simulink model "GCAWS"  (R2022a)
settings: Solver=FixedStepDiscrete  StartTime=0.0  StopTime=1  FixedStep=0.04  RelTol=1e-3
PreLoadFcn:
  | % Add Module Path
  | listing = dir;
  | if (contains([listing .name], 'TCAF')) && (contains([listing .name], 'MAP'))
  |     addpath('./TCAF', './MAP');
  |     addpath( genpath('./MAP') );
  | elseif (contains([listing .name], 'GCAWS.slx'))
  |     addpath('../TCAF', '../MAP');
  |     addpath( genpath('../MAP') );
  | else
  | end
  | 
  | % Add DataBus Path
  | load('BusStructureGCAWS.mat');
  | load('BusStructureWTPG.mat');
  | load('TRN\BusStructureTRN.mat');
InitFcn:
  | % Add Module Path
  | listing = dir;
  | if (contains([listing .name], 'TCAF')) && (contains([listing .name], 'MAP'))
  |     addpath('./TCAF', './MAP');
  |     addpath( genpath('./MAP') );
  | elseif (contains([listing .name], 'GCAWS.slx'))
  |     addpath('../TCAF', '../MAP');
  |     addpath( genpath('../MAP') );
  | else
  | end
  | 
  | % Add DataBus Path
  | load('BusStructureGCAWS.mat');
  | load('BusStructureWTPG.mat');
  | load('TRN\BusStructureTRN.mat');
StartFcn:
  | % Add Module Path
  | listing = dir;
  | if (contains([listing .name], 'TCAF')) && (contains([listing .name], 'MAP'))
  |     addpath('./TCAF', './MAP');
  |     addpath( genpath('./MAP') );
  | elseif (contains([listing .name], 'GCAWS.slx'))
  |     addpath('../TCAF', '../MAP');
  |     addpath( genpath('../MAP') );
  | else
  | end
  | 
  | % Add DataBus Path
  | load('BusStructureGCAWS.mat');
  | load('BusStructureWTPG.mat');
  | load('TRN\BusStructureTRN.mat');
values from neighbouring files (symbols this model uses):
  isFeasible = logsout{idx_WTPGDatapump}.Values.isFeasible.Data(ii,:)    [WTPG_SIM_AFTERPLOT.m]
undefined symbols (not defined in the file or in its folder): accNED, C_b_n, collisionWarning, collisionWarningValid, gOnsetRateWrap, lla, maxFlightPathAngleWrap, offObstructionMap, offTerrainMap, params, paramSelectedValid, pullUpGWrap, reactionTimeWrap, rollRateWrap, selectedWrap, statusCode, timeToGoToPullUp, velNED
libraries: hdlsllib x15, simulink x2
(part 1 of 2)
settings Model: Creator=ASCL  LastModifiedBy=ASCL
settings DataIOCC: SaveOutput=off  SignalLogging=off  DSMLogging=off  SaveTime=off  ReturnWorkspaceOutputs=off
settings OptimizationCC: BlockReduction=off  DefaultParameterBehavior=Inlined  UseDivisionForNetSlopeComputation=on  GainParamInheritBuiltInType=on  UseFloatMulNetSlope=on  ExpressionFolding=off  PassReuseOutputArgsAs=Individual arguments  ZeroExternalMemoryAtStartup=off  ZeroInternalMemoryAtStartup=off  EfficientFloat2IntCast=on  LifeSpan=inf  OptimizeBlockOrder=speed  DifferentSizesBufferReuse=on  EfficientTunableParamExpr=on
settings DebuggingCC: SignalInfNanChecking=warning  ReadBeforeWriteMsg=EnableAllAsError  WriteAfterWriteMsg=EnableAllAsError  WriteAfterReadMsg=EnableAllAsError  IntegerOverflowMsg=error  ParameterTunabilityLossMsg=error  UniqueDataStoreMsg=error  AssertControl=DisableAll  NonBusSignalsTreatedAsBus=error  SFInvalidInputDataAccessInChartInitDiag=error  SFTransitionOutsideNaturalParentDiag=error  SFUnreachableExecutionPathDiag=error  SFUndirectedBroadcastEventsDiag=error  IntegerSaturationMsg=error
settings HardwareCC: ProdBitPerPointer=32  ProdBitPerSizeT=32  ProdBitPerPtrDiffT=32  ProdLargestAtomicInteger=Long  ProdLargestAtomicFloat=Double  ProdEndianess=BigEndian  ProdWordSize=32  ProdLongLongMode=on  ProdHWDeviceType=Freescale->MPC83xx
settings ModelReferenceCC: ModelReferenceNumInstancesAllowed=Single
settings SFSimCC: SimCustomHeaderCode="#include \"MAP.h\""  SimUserSources=MAP.c  SimUserLibraries=WS2_32.LIB  CompileTimeRecursionLimit=0  EnableRuntimeRecursion=off  MATLABDynamicMemAlloc=off
settings RTWCC: SystemTargetFile=ert.tlc  TemplateMakefile=ert_default_tmf  GenerateReport=on  RTWUseSimCustomCode=on  CustomHeaderCode="#include \"MAP.h\""  CustomSource=MAP.c  CustomLibrary=WS2_32.LIB  BuildConfiguration=Faster Runs  IncludeHyperlinkInReport=on  LaunchReport=on  GenerateTraceInfo=on  GenerateTraceReport=on  GenerateTraceReportSl=on  GenerateTraceReportSf=on  GenerateTraceReportEml=on  GenerateCodeMetricsReport=on
settings CodeAppCC: ForceParamTrailComments=on  IgnoreCustomStorageClasses=off  OperatorAnnotations=on  SimulinkDataObjDesc=on  SFDataObjDesc=on  MATLABFcnDesc=on  InsertBlockDesc=on  StateflowObjectComments=on  MATLABSourceComments=on  EnableCustomComments=on  InlinedPrmAccess=Macros  ReqsInCode=on
settings ERTTargetCC: TargetLangStandard=C99 (ISO)  UtilityFuncGeneration=Shared location  GenerateSampleERTMain=on  IncludeMdlTerminateFcn=off  CombineSignalStateStructs=on  SuppressErrorStatus=on  SupportAbsoluteTime=off  SupportNonFinite=off  SupportComplex=off  SupportVariableSizeSignals=on  ParenthesesLevel=Standards  CastingMode=Standards  GenerateSharedConstants=off  InlinedParameterPlacement=NonHierarchical  ERTCustomFileTemplate=example_file_process.tlc  RateTransitionBlockCode=Function  PreserveIfCondition=on  ConvertIfToSwitch=off  EnableSignedLeftShifts=off  EnableSignedRightShifts=off

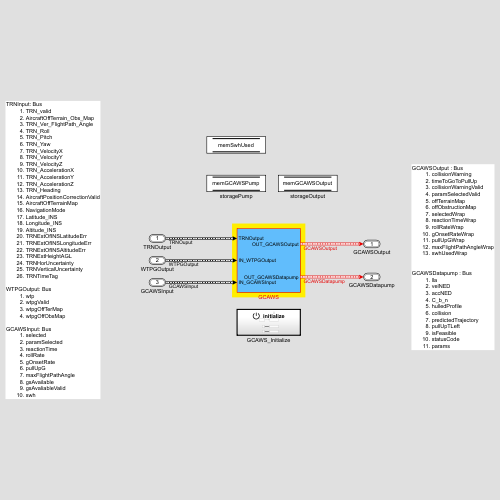
[thumbnail: Simulink's stored preview of the top-level diagram]
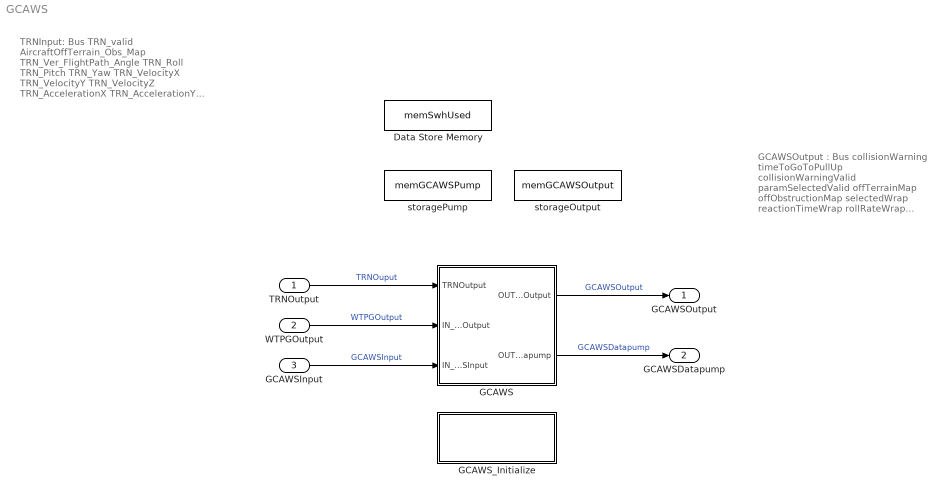
== system GCAWS ==
  note: TRNInput: Bus
      | TRN_valid
      | AircraftOffTerrain_Obs_Map
      | TRN_Ver_FlightPath_Angle
      | TRN_Roll
      | TRN_Pitch
      | TRN_Yaw
      | TRN_VelocityX
      | TRN_VelocityY
      | TRN_VelocityZ
      | TRN_AccelerationX
      | TRN_AccelerationY
      | TRN_AccelerationZ
      | TRN_Heading
      | AircraftPositionCorrectionValid
      | AircraftOffTerrainMap
      | NavigationMode
      | Latitude_INS
      | Longitude_INS
      | Altitude_INS
      | TRNEstOfINSLatitudeErr
      | TRNEstOfINSLongitudeErr
      | TRNEstOfINSAltitudeErr
      | TRNEstHeightAGL
      | TRNHorUncertainty
      | TRNVerticalUncertainty
      | TRNTimeTag
      |
      | WTPGOutput: Bus
      | wtp
      | wtpgValid
      | wtpgOffTerMap
      | wtpgOffObsMap
      |
      | GCAWSInput: Bus
      | selected
      | paramSelected
      | reactionTime
      | rollRate
      | gOnsetRate
      | pullUpG
      | maxFlightPathAngle
      | gsAvailable
      | gsAvaliableValid
      | swh
  note: GCAWSOutput : Bus
      | collisionWarning
      | timeToGoToPullUp
      | collisionWarningValid
      | paramSelectedValid
      | offTerrainMap
      | offObstructionMap
      | selectedWrap
      | reactionTimeWrap
      | rollRateWrap
      | gOnsetRateWrap
      | pullUpGWrap
      | maxFlightPathAngleWrap
      | swhUsedWrap
      |
      | GCAWSDatapump : Bus
      | lla
      | velNED
      | accNED
      | C_b_n
      | hulledProfile
      | collision
      | predictedTrajectory
      | pullUpTLeft
      | isFeasible
      | statusCode
      | params
  TRNOutput : Inport  OutDataTypeStr=Bus: TRNOutput  Interpolate=off  BusOutputAsStruct=on
  WTPGOutput : Inport  Port=2  OutDataTypeStr=Bus: WTPGOutput  Interpolate=off  BusOutputAsStruct=on
  GCAWSInput : Inport  Port=3  OutDataTypeStr=Bus: GCAWSInput  Interpolate=off  BusOutputAsStruct=on
  Data Store Memory : DataStoreMemory  DataStoreName=memSwhUsed  WriteAfterWriteMsg=warning  ShowAdditionalParam=off  OutDataTypeStr=single
  GCAWS : Subsystem
      mask init:
      | % latGPS = double(0);
      | % lonGPS = double(0);
      | % altGPS = double(0);
      | % velEGPS = double(0);
      | % velNGPS = double(0);
      | % velUGPS = double(0);
      | % notValidGPS = boolean(0);
      | % notAvaildINS = boolean(0);
      | % velUINS = double(0);
      | % velVINS = double(0);
      | % velWINS = double(0);
      | % rollINS = double(0);
      | % pitchINS = double(0);
      | % hgdINS = double(0);
      | % accXINS = double(0);
      | % accYINS = double(0);
      | % accZINS = double(0);
      | % activated = boolean(0);
      | % reactionT = uint16(0);
      | % pullUpG = uint16(0);
      | % rollRate = uint16(0);
      | % gOnsetRate = uint16(0);
      | % maxGamma = uint16(0);
      | % setWarnH = double(0);
      | % obsWarningTime = uint16(1);
      | % wiresWarningTime = uint16(1);
      | % latErrOfINS = double(0);
      | % lonErrOfINS = double(0);
      | % altErrorofINS = uint16(0);
      | % heightEstOfTRN = uint16(0);
      | % horUncertaintyOfTRN = double(0);
      | % verUncertaintyOfTRN = double(0);
  GCAWS_Initialize : Subsystem  TreatAsAtomicUnit=on
  storageOutput : DataStoreMemory  DataStoreName=memGCAWSOutput  WriteAfterWriteMsg=warning  WriteAfterReadMsg=warning  VectorParams1D=off  ShowAdditionalParam=off  OutDataTypeStr=Bus: GCAWSOutput
      settings: LockScale=on
  storagePump : DataStoreMemory  DataStoreName=memGCAWSPump  WriteAfterWriteMsg=warning  WriteAfterReadMsg=warning  VectorParams1D=off  ShowAdditionalParam=off  OutDataTypeStr=Bus: GCAWSDatapump
      settings: LockScale=on
  GCAWSOutput : Outport  OutDataTypeStr=Bus: GCAWSOutput  VectorParamsAs1DForOutWhenUnconnected=off  BusOutputAsStruct=on
  GCAWSDatapump : Outport  Port=2  OutDataTypeStr=Bus: GCAWSDatapump  VectorParamsAs1DForOutWhenUnconnected=off  BusOutputAsStruct=on
  wires:
  GCAWS/1(OUT_GCAWSOutput) -> GCAWSOutput/1  "GCAWSOutput"
  GCAWS/2(OUT_GCAWSDatapump) -> GCAWSDatapump/1  "GCAWSDatapump"
  GCAWSInput/1 -> GCAWS/3(IN_GCAWSInput)  "GCAWSInput"
  TRNOutput/1 -> GCAWS/1(TRNOutput)  "TRNOuput"
  WTPGOutput/1 -> GCAWS/2(IN_WTPGOutput)  "WTPGOutput"

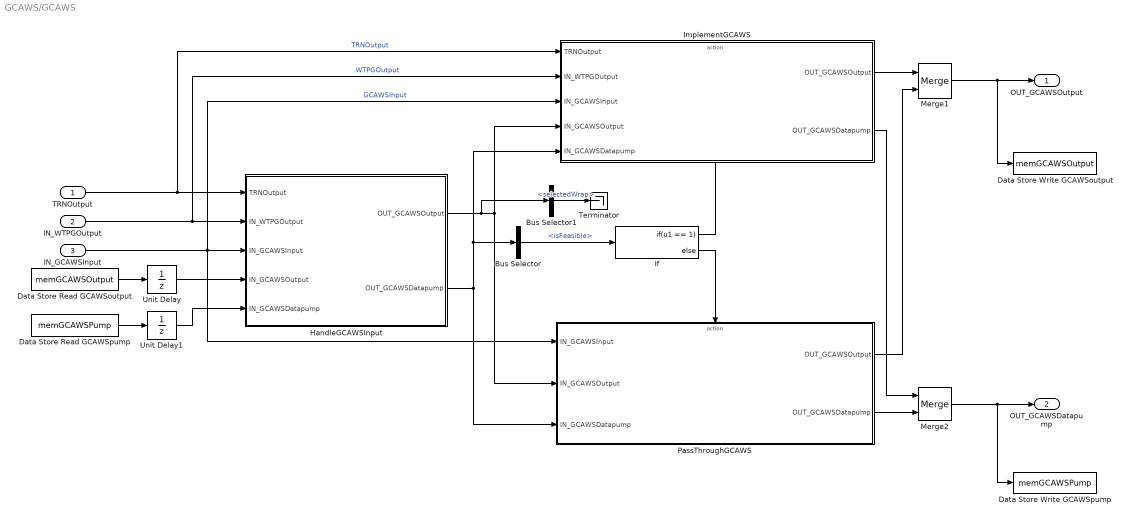
== system GCAWS/GCAWS ==
  TRNOutput : Inport  OutDataTypeStr=Bus: TRNOutput  BusOutputAsStruct=on
  IN_WTPGOutput : Inport  Port=2  OutDataTypeStr=Bus: WTPGOutput
  IN_GCAWSInput : Inport  Port=3  OutDataTypeStr=Bus: GCAWSInput
  Bus Selector : BusSelector  OutputSignals=isFeasible
  Bus Selector1 : BusSelector  OutputSignals=selectedWrap
  Data Store Read GCAWSoutput : DataStoreRead  DataStoreName=memGCAWSOutput  IndexOptions=Index vector (dialog)  Indices=1  OutputSizes=1
  Data Store Read GCAWSpump : DataStoreRead  DataStoreName=memGCAWSPump  IndexOptions=Index vector (dialog)  Indices=1  OutputSizes=1
  Data Store Write GCAWSoutput : DataStoreWrite  DataStoreName=memGCAWSOutput  IndexOptions=Index vector (dialog)  Indices=1  OutputSizes=1
  Data Store Write GCAWSpump : DataStoreWrite  DataStoreName=memGCAWSPump  IndexOptions=Index vector (dialog)  Indices=1  OutputSizes=1
  HandleGCAWSInput : Subsystem  TreatAsAtomicUnit=on
      settings: RTWSystemCode=Nonreusable function  RTWFcnNameOpts=Use subsystem name
  If : If  IfExpression=u1 == 1
  ImplementGCAWS : Subsystem  TreatAsAtomicUnit=on
      settings: RTWSystemCode=Nonreusable function  RTWFcnNameOpts=Use subsystem name
  Merge1 : Merge
  Merge2 : Merge
  PassThroughGCAWS : Subsystem  TreatAsAtomicUnit=on
      settings: RTWSystemCode=Nonreusable function  RTWFcnNameOpts=Use subsystem name
  Terminator : Terminator
  Unit Delay : UnitDelay  SampleTime=-1  HasFrameUpgradeWarning=on
  Unit Delay1 : UnitDelay  SampleTime=-1  HasFrameUpgradeWarning=on
  OUT_GCAWSOutput : Outport  OutDataTypeStr=Bus: GCAWSOutput  VectorParamsAs1DForOutWhenUnconnected=off
  OUT_GCAWSDatapump : Outport  Port=2  OutDataTypeStr=Bus: GCAWSDatapump  VectorParamsAs1DForOutWhenUnconnected=off
  wires:
  IN_GCAWSInput/1 -> ImplementGCAWS/3(IN_GCAWSInput), PassThroughGCAWS/1(IN_GCAWSInput), HandleGCAWSInput/3(IN_GCAWSInput)  "GCAWSInput"
  Merge1/1 -> Data Store Write GCAWSoutput/1, OUT_GCAWSOutput/1
  HandleGCAWSInput/1(OUT_GCAWSOutput) -> Bus Selector1/1, ImplementGCAWS/4(IN_GCAWSOutput), PassThroughGCAWS/2(IN_GCAWSOutput)
  HandleGCAWSInput/2(OUT_GCAWSDatapump) -> Bus Selector/1, ImplementGCAWS/5(IN_GCAWSDatapump), PassThroughGCAWS/3(IN_GCAWSDatapump)
  ImplementGCAWS/1(OUT_GCAWSOutput) -> Merge1/1
  PassThroughGCAWS/1(OUT_GCAWSOutput) -> Merge1/2
  PassThroughGCAWS/2(OUT_GCAWSDatapump) -> Merge2/2
  ImplementGCAWS/2(OUT_GCAWSDatapump) -> Merge2/1
  Merge2/1 -> OUT_GCAWSDatapump/1, Data Store Write GCAWSpump/1
  If/2 -> PassThroughGCAWS/Action
  If/1 -> ImplementGCAWS/Action
  IN_WTPGOutput/1 -> ImplementGCAWS/2(IN_WTPGOutput), HandleGCAWSInput/2(IN_WTPGOutput)  "WTPGOutput"
  TRNOutput/1 -> ImplementGCAWS/1(TRNOutput), HandleGCAWSInput/1(TRNOutput)  "TRNOutput"
  Bus Selector/1 -> If/1  "<isFeasible>"
  Data Store Read GCAWSoutput/1 -> Unit Delay/1
  Data Store Read GCAWSpump/1 -> Unit Delay1/1
  Unit Delay/1 -> HandleGCAWSInput/4(IN_GCAWSOutput)
  Unit Delay1/1 -> HandleGCAWSInput/5(IN_GCAWSDatapump)
  Bus Selector1/1 -> Terminator/1  "<selectedWrap>"

== system GCAWS/GCAWS_Initialize ==
  Constant : Constant  Value=[0, ]  OutDataTypeStr=Bus: GCAWSOutput
  Constant1 : Constant  Value=[0, ]  OutDataTypeStr=Bus: GCAWSDatapump
  Constant_single : Constant  Value=single(15.24)  OutDataTypeStr=single
  Data Store Write : DataStoreWrite  DataStoreName=memSwhUsed  IndexOptions=Index vector (dialog)  Indices=1  OutputSizes=1
  Data Store Write1 : DataStoreWrite  DataStoreName=memGCAWSPump  IndexOptions=Index vector (dialog)  Indices=1  OutputSizes=1
  Data Store Write2 : DataStoreWrite  DataStoreName=memGCAWSOutput  IndexOptions=Index vector (dialog)  Indices=1  OutputSizes=1
  Event Listener : EventListener  DisableCoverage=on  EventName=reset
  wires:
  Constant/1 -> Data Store Write2/1
  Constant_single/1 -> Data Store Write/1
  Constant1/1 -> Data Store Write1/1

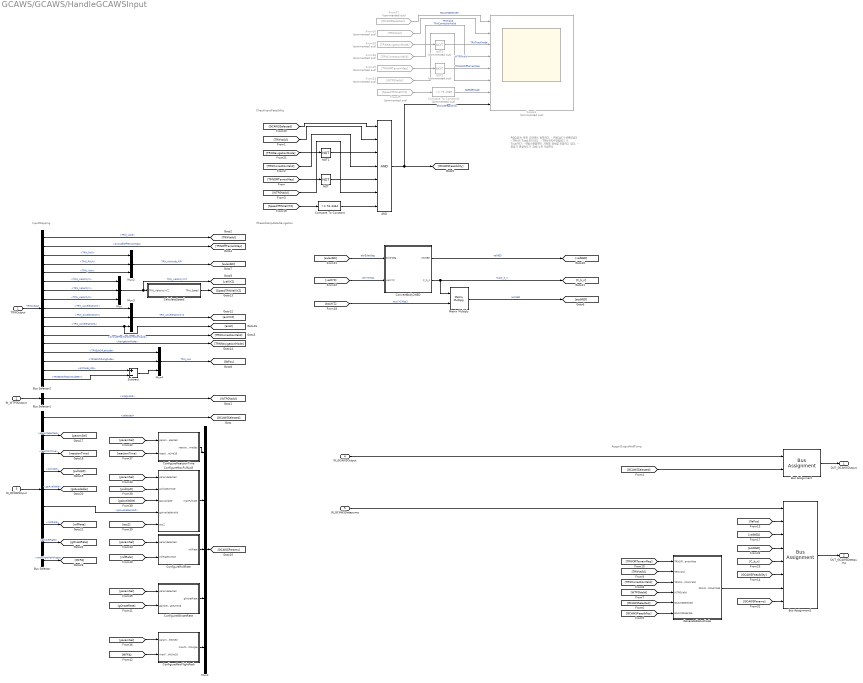
== system GCAWS/GCAWS/HandleGCAWSInput ==
  note: AssginOutputAndPump
  note: CheckInputFeasibility
  note: IfFeasibleUpdateNavigation
  note: PGCAS는 아래 조건에서 동작한다.
      | - PGCAS가 선택되었다.
      | - TRN이 Track모드이다.
      | - TRN 위치수정플래그가 True이다.
      | - 전방스캔영역의 지형맵 정보를 포함하고 있다.
      | - 항공기 관성속도가 100 노트 이상이다
  note: InputMapping
  TRNOutput : Inport  OutDataTypeStr=Bus: TRNOutput
  IN_WTPGOutput : Inport  Port=2  OutDataTypeStr=Bus: WTPGOutput
  IN_GCAWSInput : Inport  Port=3  OutDataTypeStr=Bus: GCAWSInput
  IN_GCAWSOutput : Inport  Port=4  OutDataTypeStr=Bus: GCAWSOutput
  IN_GCAWSDatapump : Inport  Port=5  OutDataTypeStr=Bus: GCAWSDatapump
  AND : Logic  Inputs=7  AllPortsSameDT=off  OutDataTypeStr=boolean
  Bus Assignment : BusAssignment  AssignedSignals=selectedWrap
  Bus Assignment1 : BusAssignment  AssignedSignals=lla,velNED,accNED,C_b_n,isFeasible,statusCode,params
  Bus Selector : BusSelector  OutputSignals=selected,paramSelected,reactionTime,pullUpG,gsAvailable,gsAvaliableValid,rollRate,gOnsetRate,maxFlightPathAngle
  Bus Selector1 : BusSelector  OutputSignals=wtpgValid
  Bus Selector2 : BusSelector  OutputSignals=TRN_valid,AircraftOffTerrainMap,TRN_Roll,TRN_Pitch,TRN_Yaw,TRN_VelocityX,TRN_VelocityY,TRN_VelocityZ,TRN_AccelerationX,TRN_AccelerationY,TRN_AccelerationZ,AircraftPositionCorrectionValid,NavigationMode,TRNEstOfLatitude,TRNEstOfLongitude,Altitude_INS,TRNEstOfINSAltitudeErr
  CalculateSpeed : Subsystem
  Compare To Constant : simulink/Logic and Bit Operations/Compare To Constant  relop=>=  const=51.4444  OutDataTypeStr=boolean
  Compare To Constant1 : simulink/Logic and Bit Operations/Compare To Constant  Commented=on  relop=>=  const=75.1089  OutDataTypeStr=boolean
  ConfigureGOnsetRate : MATLAB Function  TreatAsAtomicUnit=on
      settings: RTWSystemCode=Nonreusable function  RTWFcnNameOpts=Use subsystem name  FunctionInterfaceSpec=Allow arguments (Match graphical interface)
  ConfigureMaxFlightPath : MATLAB Function  TreatAsAtomicUnit=on
      settings: RTWSystemCode=Nonreusable function  RTWFcnNameOpts=Use subsystem name  FunctionInterfaceSpec=Allow arguments (Match graphical interface)
  ConfigureMaxPullUpG : MATLAB Function  TreatAsAtomicUnit=on
      settings: RTWSystemCode=Nonreusable function  RTWFcnNameOpts=Use subsystem name  FunctionInterfaceSpec=Allow arguments (Match graphical interface)
  ConfigureReactionTime : MATLAB Function  TreatAsAtomicUnit=on
      settings: RTWSystemCode=Nonreusable function  RTWFcnNameOpts=Use subsystem name  FunctionInterfaceSpec=Allow arguments (Match graphical interface)
  ConfigureRollRate : MATLAB Function  TreatAsAtomicUnit=on
      settings: RTWSystemCode=Nonreusable function  RTWFcnNameOpts=Use subsystem name  FunctionInterfaceSpec=Allow arguments (Match graphical interface)
  ConvertBody2NED : MATLAB Function  TreatAsAtomicUnit=on
  From15 : From  Commented=on  GotoTag=TRNOffTerrainMap
  From16 : From  Commented=on  GotoTag=TRNValid
  From25 : From  Commented=on  GotoTag=SpeedTRNVelXYZ
  From26 : From  Commented=on  GotoTag=TRNCorrectionValid
  From27 : From  Commented=on  GotoTag=GCAWSSelected
  From28 : From  Commented=on  GotoTag=TRNNavigationMode
  From29 : From  Commented=on  GotoTag=WTPGValid
  GenerateStatusCode : Subsystem
  Matrix Multiply : Product  Multiplication=Matrix(*)
  Mux{,2..4} (4 alike) : Mux  Inputs=3
  Mux1 : Mux  Inputs=5
  NOT : Logic  Operator=NOT  AllPortsSameDT=off  OutDataTypeStr=boolean
  NOT1 : Logic  Operator=NOT  AllPortsSameDT=off  OutDataTypeStr=boolean
  NOT2 : Logic  Commented=on  Operator=NOT  AllPortsSameDT=off  OutDataTypeStr=boolean
  NOT3 : Logic  Commented=on  Operator=NOT  AllPortsSameDT=off  OutDataTypeStr=boolean
  Scope1 : Scope  Commented=on  NumInputPorts=8
  Subtract : Sum  Inputs=+-
  OUT_GCAWSOutput : Outport  OutDataTypeStr=Bus: GCAWSOutput  VectorParamsAs1DForOutWhenUnconnected=off
  OUT_GCAWSDatapump : Outport  Port=2  OutDataTypeStr=Bus: GCAWSDatapump  VectorParamsAs1DForOutWhenUnconnected=off
  wires:
  IN_GCAWSDatapump/1 -> Bus Assignment1/1
  IN_GCAWSInput/1 -> Bus Selector/1
  IN_GCAWSOutput/1 -> Bus Assignment/1
  Bus Selector/1 -> [GCAWSSelected]  "<selected>"
  Bus Assignment/1 -> OUT_GCAWSOutput/1
  IN_WTPGOutput/1 -> Bus Selector1/1
  AND/1 -> [GCAWSFeasibility], Scope1/8  "GCAWSFeasibility"
  Bus Selector1/1 -> [WTPGValid]  "<wtpgValid>"
  TRNOutput/1 -> Bus Selector2/1  "TRNOutput"
  Bus Selector2/2 -> [TRNOffTerrainMap]  "<AircraftOffTerrainMap>"
  Bus Selector2/1 -> [TRNValid]  "<TRN_valid>"
  Bus Selector2/12 -> [TRNCorrectionValid]  "<AircraftPositionCorrectionValid>"
  [TRNOffTerrainMap] -> NOT/1
  [GCAWSSelected] -> Bus Assignment/2
  Bus Assignment1/1 -> OUT_GCAWSDatapump/1
  GenerateStatusCode/1(GCAWSStatusCode) -> Bus Assignment1/7
  CalculateSpeed/1(TRN_Speed) -> [SpeedTRNVelXYZ]
  [SpeedTRNVelXYZ] -> Compare To Constant/1
  [GCAWSSelected] -> AND/1
  [TRNCorrectionValid] -> AND/4
  Bus Selector2/13 -> [TRNNavigationMode]  "<NavigationMode>"
  NOT/1 -> AND/5
  [TRNValid] -> AND/2
  [TRNNavigationMode] -> NOT1/1
  [WTPGValid] -> AND/6
  Compare To Constant/1 -> AND/7
  Bus Selector2/8 -> Mux/3  "<TRN_VelocityZ>"
  Bus Selector2/7 -> Mux/2  "<TRN_VelocityY>"
  Bus Selector2/6 -> Mux/1  "<TRN_VelocityX>"
  Mux/1 -> [velXYZ], CalculateSpeed/1(TRN_VelocityXYZ)  "TRN_VelocityXYZ"
  Bus Selector2/3 -> Mux2/1  "<TRN_Roll>"
  Bus Selector2/4 -> Mux2/2  "<TRN_Pitch>"
  Bus Selector2/5 -> Mux2/3  "<TRN_Yaw>"
  Mux2/1 -> [eulerAtti]  "TRN_Attitude_RPY"
  Bus Selector2/11 -> [accZ], Mux3/3  "<TRN_AccelerationZ>"
  Bus Selector2/10 -> Mux3/2  "<TRN_AccelerationY>"
  Bus Selector2/9 -> Mux3/1  "<TRN_AccelerationX>"
  Mux3/1 -> [accXYZ]  "TRN_AccelerationXYZ"
  Bus Selector2/14 -> Mux4/1  "<TRNEstOfLatitude>"
  Bus Selector2/15 -> Mux4/2  "<TRNEstOfLongitude>"
  Bus Selector2/16 -> Subtract/1  "<Altitude_INS>"
  Bus Selector2/17 -> Subtract/2  "<TRNEstOfINSAltitudeErr>"
  Subtract/1 -> Mux4/3
  Mux4/1 -> [llaPos]  "TRN_LLA"
  [eulerAtti] -> ConvertBody2NED/1(eulerDeg)  "attiEulerDeg"
  [velXYZ] -> ConvertBody2NED/2(vecXYZ)  "velXYZMps"
  [accXYZ] -> Matrix Multiply/2  "accXYZMps2"
  ConvertBody2NED/2(C_b_n) -> Matrix Multiply/1, [C_b_n]  "matC_b_n"
  ConvertBody2NED/1(vecNED) -> [velNED]  "velNED"
  Matrix Multiply/1 -> [accNED]  "accNED"
  [velNED] -> Bus Assignment1/3
  [C_b_n] -> Bus Assignment1/5
  [accNED] -> Bus Assignment1/4
  [llaPos] -> Bus Assignment1/2
  [GCAWSFeasibility] -> Bus Assignment1/6
  [TRNOffTerrainMap] -> GenerateStatusCode/1(TRNOffTerrainMap)
  [TRNValid] -> GenerateStatusCode/2(TRNValid)
  [TRNCorrectionValid] -> GenerateStatusCode/3(TRNCorrectionValid)
  [WTPGValid] -> GenerateStatusCode/4(WTPGValid)
  [GCAWSSelected] -> GenerateStatusCode/5(GCAWSSelected)
  [GCAWSFeasibility] -> GenerateStatusCode/6(GCAWSFeasible)
  NOT1/1 -> AND/3
  NOT3/1 -> Scope1/3  "TRNTrackMode"
  From29/1 -> Scope1/6  "WTPGValid"
  From28/1 -> NOT3/1
  From16/1 -> Scope1/2  "TRNValid"
  NOT2/1 -> Scope1/5  "TRNNotOffTerrainMap"
  From26/1 -> Scope1/4  "TRNCorrectionValid"
  From27/1 -> Scope1/1  "GCAWSSelected"
  From25/1 -> Compare To Constant1/1
  From15/1 -> NOT2/1
  Compare To Constant1/1 -> Scope1/7  "SpeedEnough"
  Bus Selector/2 -> [paramSel]  "<paramSelected>"
  Bus Selector/3 -> [reactionTime]  "<reactionTime>"
  Bus Selector/7 -> [rollRate]  "<rollRate>"
  Bus Selector/8 -> [gOnsetRate]  "<gOnsetRate>"
  Bus Selector/4 -> [pullUpG]  "<pullUpG>"
  Bus Selector/9 -> [MFPA]  "<maxFlightPathAngle>"
  Bus Selector/5 -> [gsAvailable]  "<gsAvailable>"
  Bus Selector/6 -> ConfigureMaxPullUpG/4(gsAvailableValid)  "<gsAvaliableValid>"
  Mux1/1 -> [GCAWSParams]
  [accZ] -> ConfigureMaxPullUpG/5(accZ)
  [GCAWSParams] -> Bus Assignment1/8
  ConfigureReactionTime/1(reactionTimeSec) -> Mux1/1
  ConfigureMaxPullUpG/1(maxPullUpG) -> Mux1/2
  ConfigureRollRate/1(rollRate) -> Mux1/3
  [paramSel] -> ConfigureReactionTime/1(paramSelected)
  [paramSel] -> ConfigureMaxPullUpG/1(paramSelected)
  [paramSel] -> ConfigureRollRate/1(paramSelected)
  ConfigureGOnsetRate/1(gOnsetRate) -> Mux1/4
  [paramSel] -> ConfigureGOnsetRate/1(paramSelected)
  ConfigureMaxFlightPath/1(maxFlightPathAngle) -> Mux1/5
  [paramSel] -> ConfigureMaxFlightPath/1(paramSelected)
  [reactionTime] -> ConfigureReactionTime/2(reactionTimeUint16)
  [pullUpG] -> ConfigureMaxPullUpG/2(pullUpGUint16)
  [gsAvailable] -> ConfigureMaxPullUpG/3(gsAvailable)
  [rollRate] -> ConfigureRollRate/2(rollRateUint16)
  [gOnsetRate] -> ConfigureGOnsetRate/2(gOnsetRateUint16)
  [MFPA] -> ConfigureMaxFlightPath/2(maxFlightPathUint16)

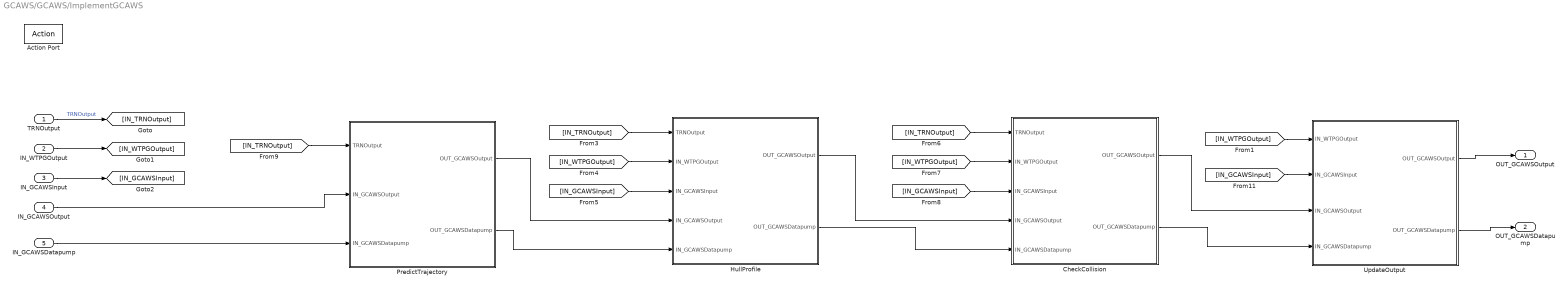
== system GCAWS/GCAWS/ImplementGCAWS ==
  TRNOutput : Inport  OutDataTypeStr=Bus: TRNOutput
  IN_WTPGOutput : Inport  Port=2  OutDataTypeStr=Bus: WTPGOutput
  IN_GCAWSInput : Inport  Port=3  OutDataTypeStr=Bus: GCAWSInput
  IN_GCAWSOutput : Inport  Port=4  OutDataTypeStr=Bus: GCAWSOutput
  IN_GCAWSDatapump : Inport  Port=5  OutDataTypeStr=Bus: GCAWSDatapump
  Action Port : ActionPort  ActionPortLabel=if(u1 == 1)
  CheckCollision : Subsystem  TreatAsAtomicUnit=on
      settings: RTWSystemCode=Nonreusable function  RTWFcnNameOpts=Use subsystem name
  HullProfile : Subsystem  TreatAsAtomicUnit=on
      settings: RTWSystemCode=Nonreusable function  RTWFcnNameOpts=Use subsystem name
  PredictTrajectory : Subsystem  TreatAsAtomicUnit=on
      settings: RTWSystemCode=Nonreusable function  RTWFcnNameOpts=Use subsystem name
  UpdateOutput : Subsystem  TreatAsAtomicUnit=on
      settings: RTWSystemCode=Nonreusable function  RTWFcnNameOpts=Use subsystem name
  OUT_GCAWSOutput : Outport  OutDataTypeStr=Bus: GCAWSOutput  VectorParamsAs1DForOutWhenUnconnected=off
  OUT_GCAWSDatapump : Outport  Port=2  OutDataTypeStr=Bus: GCAWSDatapump  VectorParamsAs1DForOutWhenUnconnected=off
  wires:
  IN_GCAWSOutput/1 -> PredictTrajectory/2(IN_GCAWSOutput)
  IN_GCAWSDatapump/1 -> PredictTrajectory/3(IN_GCAWSDatapump)
  TRNOutput/1 -> [IN_TRNOutput]  "TRNOutput"
  IN_WTPGOutput/1 -> [IN_WTPGOutput]
  IN_GCAWSInput/1 -> [IN_GCAWSInput]
  [IN_GCAWSInput] -> HullProfile/3(IN_GCAWSInput)
  [IN_WTPGOutput] -> HullProfile/2(IN_WTPGOutput)
  [IN_TRNOutput] -> HullProfile/1(TRNOutput)
  [IN_TRNOutput] -> CheckCollision/1(TRNOutput)
  [IN_WTPGOutput] -> CheckCollision/2(IN_WTPGOutput)
  [IN_GCAWSInput] -> CheckCollision/3(IN_GCAWSInput)
  HullProfile/1(OUT_GCAWSOutput) -> CheckCollision/4(IN_GCAWSOutput)
  HullProfile/2(OUT_GCAWSDatapump) -> CheckCollision/5(IN_GCAWSDatapump)
  PredictTrajectory/1(OUT_GCAWSOutput) -> HullProfile/4(IN_GCAWSOutput)
  PredictTrajectory/2(OUT_GCAWSDatapump) -> HullProfile/5(IN_GCAWSDatapump)
  [IN_TRNOutput] -> PredictTrajectory/1(TRNOutput)
  CheckCollision/1(OUT_GCAWSOutput) -> UpdateOutput/3(IN_GCAWSOutput)
  CheckCollision/2(OUT_GCAWSDatapump) -> UpdateOutput/4(IN_GCAWSDatapump)
  [IN_GCAWSInput] -> UpdateOutput/2(IN_GCAWSInput)
  UpdateOutput/2(OUT_GCAWSDatapump) -> OUT_GCAWSDatapump/1
  UpdateOutput/1(OUT_GCAWSOutput) -> OUT_GCAWSOutput/1
  [IN_WTPGOutput] -> UpdateOutput/1(IN_WTPGOutput)

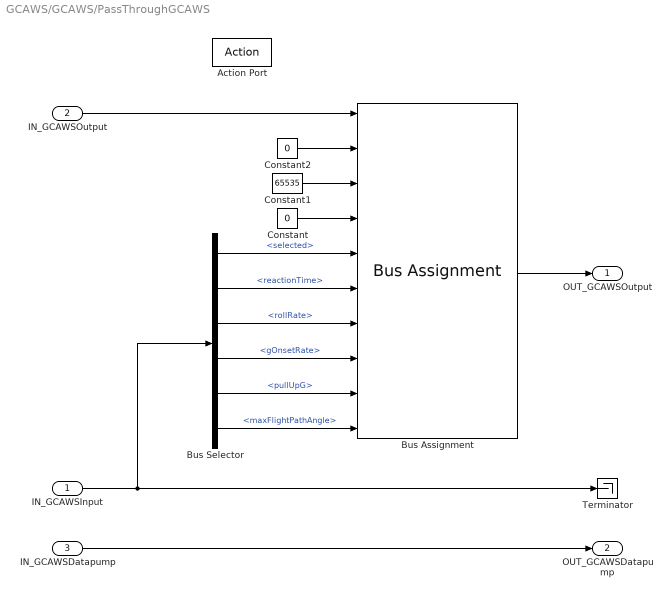
== system GCAWS/GCAWS/PassThroughGCAWS ==
  IN_GCAWSInput : Inport  OutDataTypeStr=Bus: GCAWSInput
  IN_GCAWSOutput : Inport  Port=2  OutDataTypeStr=Bus: GCAWSOutput
  IN_GCAWSDatapump : Inport  Port=3  OutDataTypeStr=Bus: GCAWSDatapump
  Action Port : ActionPort  ActionPortLabel=else
  Bus Assignment : BusAssignment  AssignedSignals=collisionWarning,timeToGoToPullUp,collisionWarningValid,selectedWrap,reactionTimeWrap,rollRateWrap,gOnsetRateWrap,pullUpGWrap,maxFlightPathAngleWrap
  Bus Selector : BusSelector  OutputSignals=selected,reactionTime,rollRate,gOnsetRate,pullUpG,maxFlightPathAngle
  Constant : Constant  Value=0  OutDataTypeStr=boolean
  Constant1 : Constant  Value=65535  OutDataTypeStr=single
  Constant2 : Constant  Value=0  OutDataTypeStr=boolean
  Terminator : Terminator
  OUT_GCAWSOutput : Outport  OutDataTypeStr=Bus: GCAWSOutput  VectorParamsAs1DForOutWhenUnconnected=off
  OUT_GCAWSDatapump : Outport  Port=2  OutDataTypeStr=Bus: GCAWSDatapump  VectorParamsAs1DForOutWhenUnconnected=off
  wires:
  Bus Selector/1 -> Bus Assignment/5  "<selected>"
  Bus Assignment/1 -> OUT_GCAWSOutput/1
  Constant/1 -> Bus Assignment/4
  IN_GCAWSInput/1 -> Bus Selector/1, Terminator/1
  IN_GCAWSDatapump/1 -> OUT_GCAWSDatapump/1
  IN_GCAWSOutput/1 -> Bus Assignment/1
  Bus Selector/6 -> Bus Assignment/10  "<maxFlightPathAngle>"
  Bus Selector/2 -> Bus Assignment/6  "<reactionTime>"
  Bus Selector/3 -> Bus Assignment/7  "<rollRate>"
  Bus Selector/4 -> Bus Assignment/8  "<gOnsetRate>"
  Bus Selector/5 -> Bus Assignment/9  "<pullUpG>"
  Constant2/1 -> Bus Assignment/2
  Constant1/1 -> Bus Assignment/3

== system GCAWS/GCAWS/HandleGCAWSInput/CalculateSpeed ==
  TRN_VelocityXYZ : Inport
  Add : Sum  Inputs=+++
  Demux : Demux  Outputs=3
  Sqrt : Sqrt
  Square : Math  Operator=square  SignedPower=on  RndMeth=Zero
  Square1 : Math  Operator=square  SignedPower=on  RndMeth=Zero
  Square2 : Math  Operator=square  SignedPower=on  RndMeth=Zero
  TRN_Speed : Outport
  wires:
  Demux/1 -> Square/1  "TRN_VelocityX"
  Demux/3 -> Square2/1  "TRN_VelocityZ"
  Demux/2 -> Square1/1  "TRN_VelocityY"
  Square/1 -> Add/1
  Square1/1 -> Add/2
  Square2/1 -> Add/3
  Add/1 -> Sqrt/1
  Sqrt/1 -> TRN_Speed/1
  TRN_VelocityXYZ/1 -> Demux/1

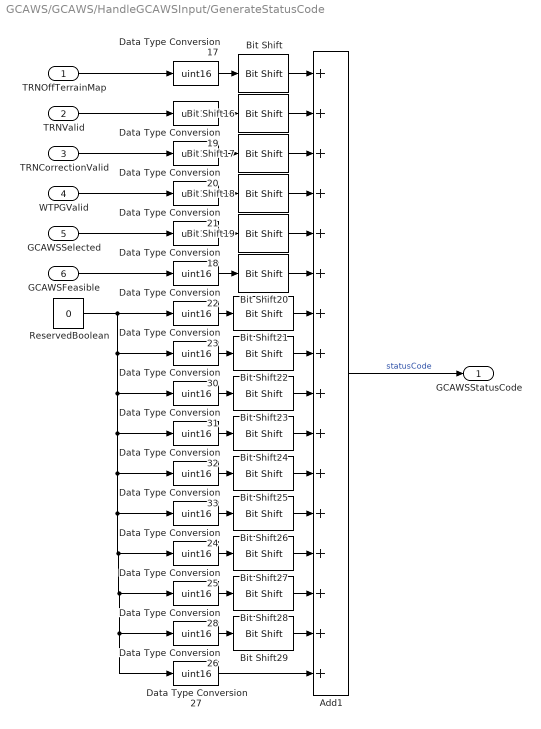
== system GCAWS/GCAWS/HandleGCAWSInput/GenerateStatusCode ==
  TRNOffTerrainMap : Inport
  TRNValid : Inport  Port=2
  TRNCorrectionValid : Inport  Port=3
  WTPGValid : Inport  Port=4
  GCAWSSelected : Inport  Port=5
  GCAWSFeasible : Inport  Port=6
  Add1 : Sum  Inputs=++++++++++++++++  AccumDataTypeStr=uint16
  Bit Shift : hdlsllib/Logic and Bit Operations/Bit Shift  mode=Shift Left Logical  N=15
  Bit Shift16 : hdlsllib/Logic and Bit Operations/Bit Shift  mode=Shift Left Logical  N=14
  Bit Shift17 : hdlsllib/Logic and Bit Operations/Bit Shift  mode=Shift Left Logical  N=13
  Bit Shift18 : hdlsllib/Logic and Bit Operations/Bit Shift  mode=Shift Left Logical  N=12
  Bit Shift19 : hdlsllib/Logic and Bit Operations/Bit Shift  mode=Shift Left Logical  N=11
  Bit Shift20 : hdlsllib/Logic and Bit Operations/Bit Shift  mode=Shift Left Logical  N=10
  Bit Shift21 : hdlsllib/Logic and Bit Operations/Bit Shift  mode=Shift Left Logical  N=9
  Bit Shift22 : hdlsllib/Logic and Bit Operations/Bit Shift  mode=Shift Left Logical  N=8
  Bit Shift23 : hdlsllib/Logic and Bit Operations/Bit Shift  mode=Shift Left Logical  N=7
  Bit Shift24 : hdlsllib/Logic and Bit Operations/Bit Shift  mode=Shift Left Logical  N=6
  Bit Shift25 : hdlsllib/Logic and Bit Operations/Bit Shift  mode=Shift Left Logical  N=5
  Bit Shift26 : hdlsllib/Logic and Bit Operations/Bit Shift  mode=Shift Left Logical  N=4
  Bit Shift27 : hdlsllib/Logic and Bit Operations/Bit Shift  mode=Shift Left Logical  N=3
  Bit Shift28 : hdlsllib/Logic and Bit Operations/Bit Shift  mode=Shift Left Logical  N=2
  Bit Shift29 : hdlsllib/Logic and Bit Operations/Bit Shift  mode=Shift Left Logical  N=1
  Data Type Conversion{17..28,30..33} (16 alike) : DataTypeConversion  OutDataTypeStr=uint16  SaturateOnIntegerOverflow=off  RndMeth=Floor
  ReservedBoolean : Constant  Value=0  OutDataTypeStr=boolean
  GCAWSStatusCode : Outport
  wires:
  Data Type Conversion28/1 -> Bit Shift28/1
  Bit Shift/1 -> Add1/1
  Data Type Conversion31/1 -> Bit Shift23/1
  Bit Shift28/1 -> Add1/14
  Data Type Conversion25/1 -> Bit Shift27/1
  Data Type Conversion27/1 -> Add1/16
  Bit Shift27/1 -> Add1/13
  Bit Shift16/1 -> Add1/2
  Data Type Conversion17/1 -> Bit Shift/1
  Bit Shift22/1 -> Add1/8
  Data Type Conversion30/1 -> Bit Shift22/1
  Data Type Conversion22/1 -> Bit Shift20/1
  Data Type Conversion32/1 -> Bit Shift24/1
  Bit Shift26/1 -> Add1/12
  Bit Shift29/1 -> Add1/15
  Bit Shift24/1 -> Add1/10
  Bit Shift25/1 -> Add1/11
  Bit Shift21/1 -> Add1/7
  Bit Shift19/1 -> Add1/5
  Bit Shift18/1 -> Add1/4
  Data Type Conversion19/1 -> Bit Shift16/1
  Bit Shift17/1 -> Add1/3
  Bit Shift20/1 -> Add1/6
  Data Type Conversion21/1 -> Bit Shift18/1
  Data Type Conversion20/1 -> Bit Shift17/1
  Data Type Conversion18/1 -> Bit Shift19/1
  Data Type Conversion24/1 -> Bit Shift26/1
  Data Type Conversion33/1 -> Bit Shift25/1
  Data Type Conversion26/1 -> Bit Shift29/1
  Bit Shift23/1 -> Add1/9
  ReservedBoolean/1 -> Data Type Conversion27/1, Data Type Conversion26/1, Data Type Conversion28/1, Data Type Conversion25/1, Data Type Conversion24/1, Data Type Conversion33/1, Data Type Conversion32/1, Data Type Conversion31/1, Data Type Conversion30/1, Data Type Conversion23/1
  Data Type Conversion23/1 -> Bit Shift21/1
  Add1/1 -> GCAWSStatusCode/1  "statusCode"
  TRNOffTerrainMap/1 -> Data Type Conversion17/1
  TRNValid/1 -> Data Type Conversion19/1
  TRNCorrectionValid/1 -> Data Type Conversion20/1
  WTPGValid/1 -> Data Type Conversion21/1
  GCAWSFeasible/1 -> Data Type Conversion22/1
  GCAWSSelected/1 -> Data Type Conversion18/1

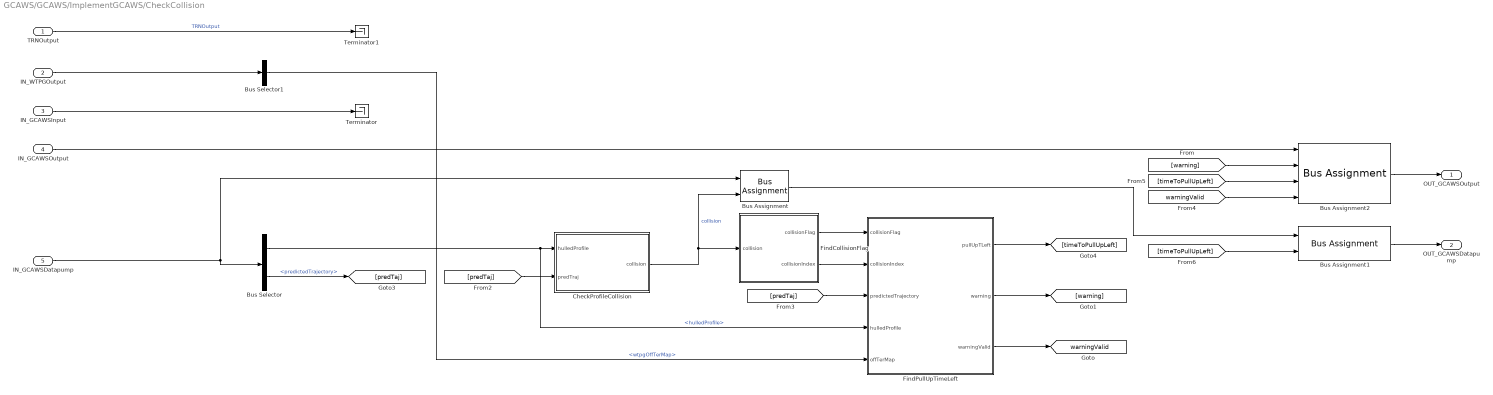
== system GCAWS/GCAWS/ImplementGCAWS/CheckCollision ==
  TRNOutput : Inport  OutDataTypeStr=Bus: TRNOutput
  IN_WTPGOutput : Inport  Port=2  OutDataTypeStr=Bus: WTPGOutput
  IN_GCAWSInput : Inport  Port=3  OutDataTypeStr=Bus: GCAWSInput
  IN_GCAWSOutput : Inport  Port=4  OutDataTypeStr=Bus: GCAWSOutput
  IN_GCAWSDatapump : Inport  Port=5  OutDataTypeStr=Bus: GCAWSDatapump
  Bus Assignment : BusAssignment  AssignedSignals=collision
  Bus Assignment1 : BusAssignment  AssignedSignals=pullUpTLeft
  Bus Assignment2 : BusAssignment  AssignedSignals=collisionWarning,timeToGoToPullUp,collisionWarningValid
  Bus Selector : BusSelector  OutputSignals=hulledProfile,predictedTrajectory
  Bus Selector1 : BusSelector  OutputSignals=wtpgOffTerMap
  CheckProfileCollision : MATLAB Function  TreatAsAtomicUnit=on
  FindCollisionFlag : MATLAB Function  TreatAsAtomicUnit=on
      settings: RTWSystemCode=Nonreusable function  RTWFcnNameOpts=Use subsystem name  FunctionInterfaceSpec=Allow arguments (Match graphical interface)
  FindPullUpTimeLeft : Subsystem
  Terminator : Terminator
  Terminator1 : Terminator
  OUT_GCAWSOutput : Outport  OutDataTypeStr=Bus: GCAWSOutput  VectorParamsAs1DForOutWhenUnconnected=off
  OUT_GCAWSDatapump : Outport  Port=2  OutDataTypeStr=Bus: GCAWSDatapump  VectorParamsAs1DForOutWhenUnconnected=off
  tag scope: warningValid=global
  wires:
  FindPullUpTimeLeft/3(warningValid) -> [warningValid]
  IN_GCAWSDatapump/1 -> Bus Assignment/1, Bus Selector/1
  CheckProfileCollision/1(collision) -> Bus Assignment/2, FindCollisionFlag/1(collision)  "collision"
  Bus Selector/1 -> FindPullUpTimeLeft/4(hulledProfile), CheckProfileCollision/1(hulledProfile)  "<hulledProfile>"
  Bus Selector/2 -> [predTaj]  "<predictedTrajectory>"
  FindCollisionFlag/1(collisionFlag) -> FindPullUpTimeLeft/1(collisionFlag)
  FindCollisionFlag/2(collisionIndex) -> FindPullUpTimeLeft/2(collisionIndex)
  Bus Assignment1/1 -> OUT_GCAWSDatapump/1
  FindPullUpTimeLeft/1(pullUpTLeft) -> [timeToPullUpLeft]
  Bus Assignment/1 -> Bus Assignment1/1
  [predTaj] -> CheckProfileCollision/2(predTraj)
  [predTaj] -> FindPullUpTimeLeft/3(predictedTrajectory)
  IN_GCAWSOutput/1 -> Bus Assignment2/1
  Bus Assignment2/1 -> OUT_GCAWSOutput/1
  [warningValid] -> Bus Assignment2/4
  [timeToPullUpLeft] -> Bus Assignment2/3
  [timeToPullUpLeft] -> Bus Assignment1/2
  IN_GCAWSInput/1 -> Terminator/1
  TRNOutput/1 -> Terminator1/1  "TRNOutput"
  FindPullUpTimeLeft/2(warning) -> [warning]
  [warning] -> Bus Assignment2/2
  IN_WTPGOutput/1 -> Bus Selector1/1
  Bus Selector1/1 -> FindPullUpTimeLeft/5(offTerMap)  "<wtpgOffTerMap>"

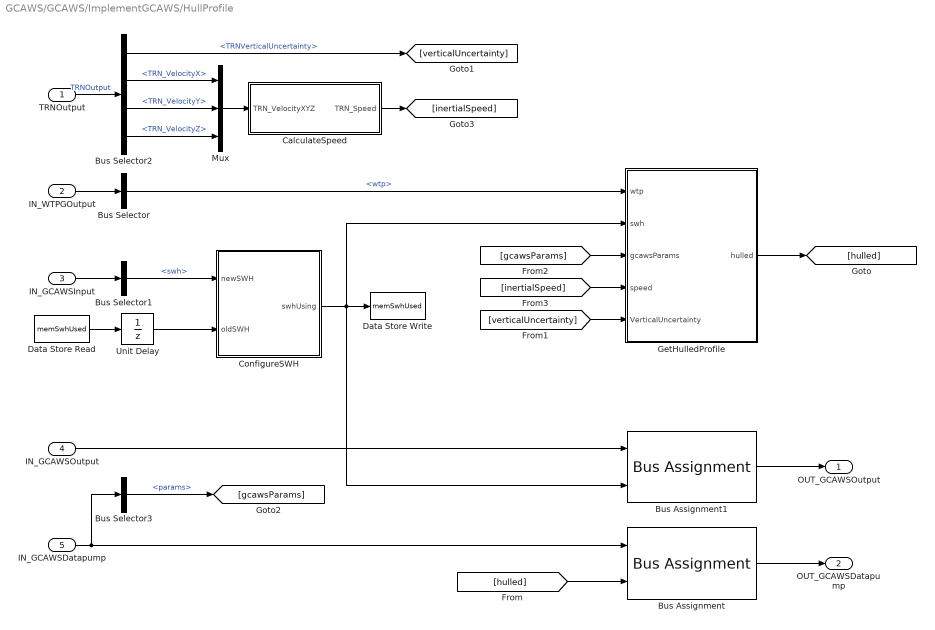
== system GCAWS/GCAWS/ImplementGCAWS/HullProfile ==
  TRNOutput : Inport  OutDataTypeStr=Bus: TRNOutput
  IN_WTPGOutput : Inport  Port=2  OutDataTypeStr=Bus: WTPGOutput
  IN_GCAWSInput : Inport  Port=3  OutDataTypeStr=Bus: GCAWSInput
  IN_GCAWSOutput : Inport  Port=4  OutDataTypeStr=Bus: GCAWSOutput
  IN_GCAWSDatapump : Inport  Port=5  OutDataTypeStr=Bus: GCAWSDatapump
  Bus Assignment : BusAssignment  AssignedSignals=hulledProfile
  Bus Assignment1 : BusAssignment  AssignedSignals=swhUsedWrap
  Bus Selector : BusSelector  OutputSignals=wtp
  Bus Selector1 : BusSelector  OutputSignals=swh
  Bus Selector2 : BusSelector  OutputSignals=TRNVerticalUncertainty,TRN_VelocityX,TRN_VelocityY,TRN_VelocityZ
  Bus Selector3 : BusSelector  OutputSignals=params
  CalculateSpeed : Subsystem
  ConfigureSWH : MATLAB Function  TreatAsAtomicUnit=on
  Data Store Read : DataStoreRead  DataStoreName=memSwhUsed  IndexOptions=Index vector (dialog)  Indices=1  OutputSizes=1
  Data Store Write : DataStoreWrite  DataStoreName=memSwhUsed  IndexOptions=Index vector (dialog)  Indices=1  OutputSizes=1
  GetHulledProfile : MATLAB Function  TreatAsAtomicUnit=on
  Mux : Mux  Inputs=3
  Unit Delay : UnitDelay  SampleTime=-1  HasFrameUpgradeWarning=on
  OUT_GCAWSOutput : Outport  OutDataTypeStr=Bus: GCAWSOutput
  OUT_GCAWSDatapump : Outport  Port=2  OutDataTypeStr=Bus: GCAWSDatapump
  wires:
  IN_WTPGOutput/1 -> Bus Selector/1
  IN_GCAWSInput/1 -> Bus Selector1/1
  Bus Selector/1 -> GetHulledProfile/1(wtp)  "<wtp>"
  TRNOutput/1 -> Bus Selector2/1  "TRNOutput"
  IN_GCAWSDatapump/1 -> Bus Assignment/1, Bus Selector3/1
  IN_GCAWSOutput/1 -> Bus Assignment1/1
  Bus Assignment/1 -> OUT_GCAWSDatapump/1
  GetHulledProfile/1(hulled) -> [hulled]
  [hulled] -> Bus Assignment/2
  Unit Delay/1 -> ConfigureSWH/2(oldSWH)
  Data Store Read/1 -> Unit Delay/1
  Bus Selector1/1 -> ConfigureSWH/1(newSWH)  "<swh>"
  ConfigureSWH/1(swhUsing) -> Bus Assignment1/2, Data Store Write/1, GetHulledProfile/2(swh)
  Bus Assignment1/1 -> OUT_GCAWSOutput/1
  Bus Selector2/1 -> [verticalUncertainty]  "<TRNVerticalUncertainty>"
  [verticalUncertainty] -> GetHulledProfile/5(VerticalUncertainty)
  Bus Selector3/1 -> [gcawsParams]  "<params>"
  [gcawsParams] -> GetHulledProfile/3(gcawsParams)
  Bus Selector2/4 -> Mux/3  "<TRN_VelocityZ>"
  Bus Selector2/3 -> Mux/2  "<TRN_VelocityY>"
  Bus Selector2/2 -> Mux/1  "<TRN_VelocityX>"
  Mux/1 -> CalculateSpeed/1(TRN_VelocityXYZ)
  CalculateSpeed/1(TRN_Speed) -> [inertialSpeed]
  [inertialSpeed] -> GetHulledProfile/4(speed)

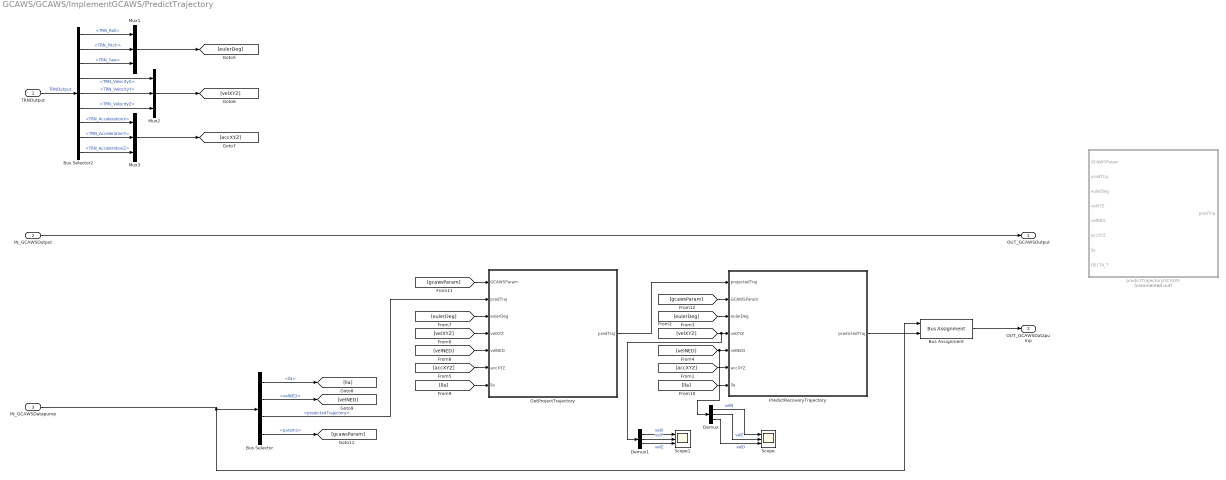
== system GCAWS/GCAWS/ImplementGCAWS/PredictTrajectory ==
  TRNOutput : Inport  OutDataTypeStr=Bus: TRNOutput
  IN_GCAWSOutput : Inport  Port=2  OutDataTypeStr=Bus: GCAWSOutput
  IN_GCAWSDatapump : Inport  Port=3  OutDataTypeStr=Bus: GCAWSDatapump
  Bus Assignment : BusAssignment  AssignedSignals=predictedTrajectory
  Bus Selector : BusSelector  OutputSignals=lla,velNED,predictedTrajectory,params
  Bus Selector2 : BusSelector  OutputSignals=TRN_Roll,TRN_Pitch,TRN_Yaw,TRN_VelocityX,TRN_VelocityY,TRN_VelocityZ,TRN_AccelerationX,TRN_AccelerationY,TRN_AccelerationZ
  Demux : Demux  Outputs=3
  Demux1 : Demux  Outputs=3
  GetProjectTrajectory : MATLAB Function
  Mux1 : Mux  Inputs=3
  Mux2 : Mux  Inputs=3
  Mux3 : Mux  Inputs=3
  PredictRecoveryTrajectory : Subsystem  TreatAsAtomicUnit=on
  Scope : Scope  NumInputPorts=3
  Scope1 : Scope  NumInputPorts=3
  predictTrajectoryGCAWS : MATLAB Function  Commented=on
  OUT_GCAWSOutput : Outport  OutDataTypeStr=Bus: GCAWSOutput
  OUT_GCAWSDatapump : Outport  Port=2  OutDataTypeStr=Bus: GCAWSDatapump  VectorParamsAs1DForOutWhenUnconnected=off
  wires:
  Bus Assignment/1 -> OUT_GCAWSDatapump/1
  PredictRecoveryTrajectory/1(predictedTraj) -> Bus Assignment/2
  IN_GCAWSDatapump/1 -> Bus Assignment/1, Bus Selector/1
  TRNOutput/1 -> Bus Selector2/1  "TRNOutput"
  Bus Selector2/1 -> Mux1/1  "<TRN_Roll>"
  Bus Selector2/2 -> Mux1/2  "<TRN_Pitch>"
  Bus Selector2/3 -> Mux1/3  "<TRN_Yaw>"
  Bus Selector2/9 -> Mux3/3  "<TRN_AccelerationZ>"
  Bus Selector2/7 -> Mux3/1  "<TRN_AccelerationX>"
  Bus Selector2/8 -> Mux3/2  "<TRN_AccelerationY>"
  Bus Selector2/5 -> Mux2/2  "<TRN_VelocityY>"
  Bus Selector2/4 -> Mux2/1  "<TRN_VelocityX>"
  Bus Selector2/6 -> Mux2/3  "<TRN_VelocityZ>"
  Mux1/1 -> [eulerDeg]
  Mux2/1 -> [velXYZ]
  Mux3/1 -> [accXYZ]
  Bus Selector/2 -> [velNED]  "<velNED>"
  Bus Selector/1 -> [lla]  "<lla>"
  IN_GCAWSOutput/1 -> OUT_GCAWSOutput/1
  Bus Selector/4 -> [gcawsParam]  "<params>"
  Bus Selector/3 -> GetProjectTrajectory/2("predTraj ")  "<predictedTrajectory>"
  [gcawsParam] -> GetProjectTrajectory/1(GCAWSParam)
  [eulerDeg] -> GetProjectTrajectory/3(eulerDeg)
  [velXYZ] -> GetProjectTrajectory/4(velXYZ)
  [velNED] -> GetProjectTrajectory/5(velNED)
  [accXYZ] -> GetProjectTrajectory/6(accXYZ)
  [lla] -> GetProjectTrajectory/7(lla)
  GetProjectTrajectory/1(predTraj) -> PredictRecoveryTrajectory/1(projectedTraj)
  [gcawsParam] -> PredictRecoveryTrajectory/2(GCAWSParam)
  [eulerDeg] -> PredictRecoveryTrajectory/3(eulerDeg)
  [velXYZ] -> Demux1/1, PredictRecoveryTrajectory/4(velXYZ)
  [velNED] -> Demux/1, PredictRecoveryTrajectory/5(velNED)
  [accXYZ] -> PredictRecoveryTrajectory/6(accXYZ)
  [lla] -> PredictRecoveryTrajectory/7(lla)
  Demux/1 -> Scope/1  "velN"
  Demux/2 -> Scope/2  "velE"
  Demux/3 -> Scope/3  "velD"
  Demux1/1 -> Scope1/1  "velX"
  Demux1/2 -> Scope1/2  "velY"
  Demux1/3 -> Scope1/3  "velZ"

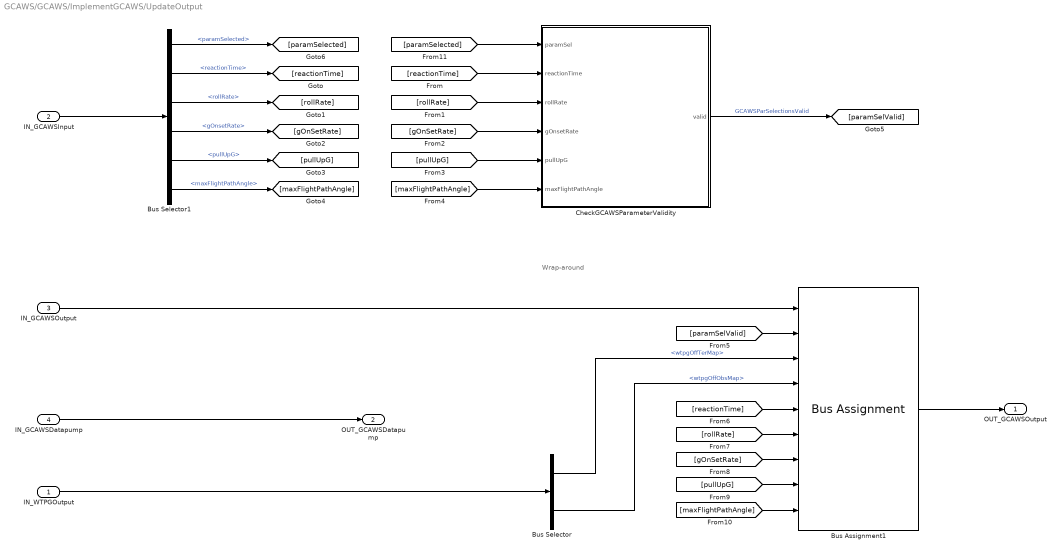
== system GCAWS/GCAWS/ImplementGCAWS/UpdateOutput ==
  note: Wrap-around
  IN_WTPGOutput : Inport  OutDataTypeStr=Bus: WTPGOutput
  IN_GCAWSInput : Inport  Port=2  OutDataTypeStr=Bus: GCAWSInput
  IN_GCAWSOutput : Inport  Port=3  OutDataTypeStr=Bus: GCAWSOutput
  IN_GCAWSDatapump : Inport  Port=4  OutDataTypeStr=Bus: GCAWSDatapump
  Bus Assignment1 : BusAssignment  AssignedSignals=paramSelectedValid,offTerrainMap,offObstructionMap,reactionTimeWrap,rollRateWrap,gOnsetRateWrap,pullUpGWrap,maxFlightPathAngleWrap
  Bus Selector : BusSelector  OutputSignals=wtpgOffTerMap,wtpgOffObsMap
  Bus Selector1 : BusSelector  OutputSignals=paramSelected,reactionTime,rollRate,gOnsetRate,pullUpG,maxFlightPathAngle
  CheckGCAWSParameterValidity : MATLAB Function  TreatAsAtomicUnit=on
      settings: RTWSystemCode=Nonreusable function  RTWFcnNameOpts=Use subsystem name  FunctionInterfaceSpec=Allow arguments (Match graphical interface)
  OUT_GCAWSOutput : Outport  OutDataTypeStr=Bus: GCAWSOutput  VectorParamsAs1DForOutWhenUnconnected=off
  OUT_GCAWSDatapump : Outport  Port=2  OutDataTypeStr=Bus: GCAWSDatapump  VectorParamsAs1DForOutWhenUnconnected=off
  wires:
  IN_GCAWSInput/1 -> Bus Selector1/1
  IN_GCAWSDatapump/1 -> OUT_GCAWSDatapump/1
  IN_GCAWSOutput/1 -> Bus Assignment1/1
  Bus Assignment1/1 -> OUT_GCAWSOutput/1
  Bus Selector1/2 -> [reactionTime]  "<reactionTime>"
  Bus Selector1/3 -> [rollRate]  "<rollRate>"
  Bus Selector1/4 -> [gOnSetRate]  "<gOnsetRate>"
  Bus Selector1/5 -> [pullUpG]  "<pullUpG>"
  Bus Selector1/6 -> [maxFlightPathAngle]  "<maxFlightPathAngle>"
  [maxFlightPathAngle] -> CheckGCAWSParameterValidity/6(maxFlightPathAngle)
  [pullUpG] -> CheckGCAWSParameterValidity/5(pullUpG)
  [gOnSetRate] -> CheckGCAWSParameterValidity/4(gOnsetRate)
  [rollRate] -> CheckGCAWSParameterValidity/3(rollRate)
  [reactionTime] -> CheckGCAWSParameterValidity/2(reactionTime)
  CheckGCAWSParameterValidity/1(valid) -> [paramSelValid]  "GCAWSParSelectionsValid"
  [paramSelValid] -> Bus Assignment1/2
  [maxFlightPathAngle] -> Bus Assignment1/9
  [pullUpG] -> Bus Assignment1/8
  [gOnSetRate] -> Bus Assignment1/7
  [rollRate] -> Bus Assignment1/6
  [reactionTime] -> Bus Assignment1/5
  IN_WTPGOutput/1 -> Bus Selector/1
  Bus Selector/1 -> Bus Assignment1/3  "<wtpgOffTerMap>"
  Bus Selector/2 -> Bus Assignment1/4  "<wtpgOffObsMap>"
  Bus Selector1/1 -> [paramSelected]  "<paramSelected>"
  [paramSelected] -> CheckGCAWSParameterValidity/1(paramSel)

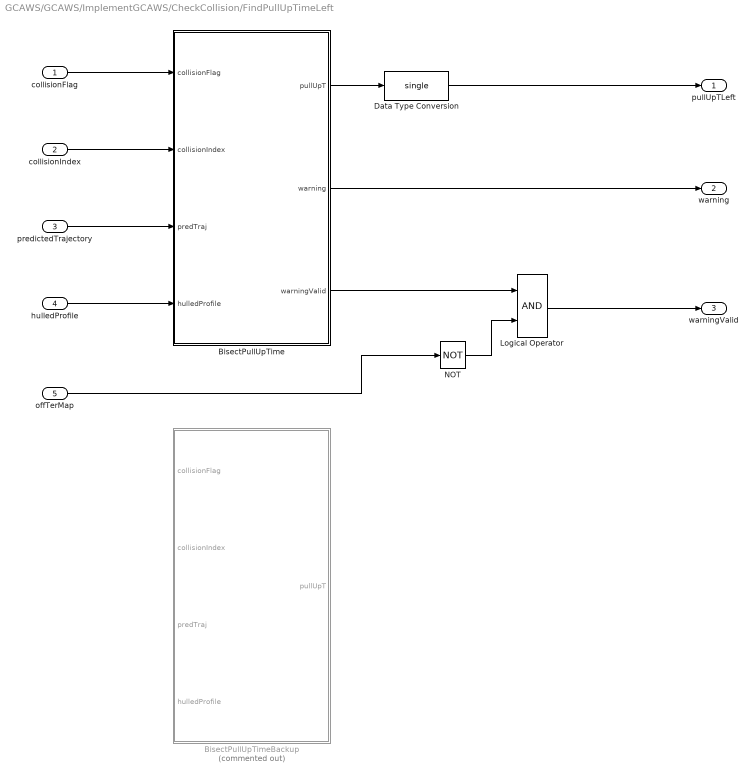
== system GCAWS/GCAWS/ImplementGCAWS/CheckCollision/FindPullUpTimeLeft ==
  collisionFlag : Inport
  collisionIndex : Inport  Port=2
  predictedTrajectory : Inport  Port=3
  hulledProfile : Inport  Port=4
  offTerMap : Inport  Port=5
  BisectPullUpTime : MATLAB Function  TreatAsAtomicUnit=on
      settings: RTWSystemCode=Nonreusable function  RTWFcnNameOpts=Use subsystem name  FunctionInterfaceSpec=Allow arguments (Match graphical interface)
  BisectPullUpTimeBackup : MATLAB Function  Commented=on  TreatAsAtomicUnit=on
      settings: RTWSystemCode=Nonreusable function  RTWFcnNameOpts=Use subsystem name  FunctionInterfaceSpec=Allow arguments (Match graphical interface)
  Data Type Conversion : DataTypeConversion  OutDataTypeStr=single  SaturateOnIntegerOverflow=off  RndMeth=Floor
  Logical Operator : Logic  AllPortsSameDT=off  OutDataTypeStr=boolean
  NOT : Logic  Operator=NOT  IconShape=distinctive  AllPortsSameDT=off  OutDataTypeStr=boolean
  pullUpTLeft : Outport  VectorParamsAs1DForOutWhenUnconnected=off
  warning : Outport  Port=2
  warningValid : Outport  Port=3  VectorParamsAs1DForOutWhenUnconnected=off
  wires:
  BisectPullUpTime/1(pullUpT) -> Data Type Conversion/1
  collisionIndex/1 -> BisectPullUpTime/2(collisionIndex)
  predictedTrajectory/1 -> BisectPullUpTime/3(predTraj)
  collisionFlag/1 -> BisectPullUpTime/1(collisionFlag)
  Data Type Conversion/1 -> pullUpTLeft/1
  Logical Operator/1 -> warningValid/1
  hulledProfile/1 -> BisectPullUpTime/4(hulledProfile)
  offTerMap/1 -> NOT/1
  BisectPullUpTime/2(warning) -> warning/1
  NOT/1 -> Logical Operator/2
  BisectPullUpTime/3(warningValid) -> Logical Operator/1

== system GCAWS/GCAWS/ImplementGCAWS/HullProfile/CalculateSpeed ==
  TRN_VelocityXYZ : Inport
  Add : Sum  Inputs=+++
  Demux : Demux  Outputs=3
  Sqrt : Sqrt
  Square : Math  Operator=square  SignedPower=on  RndMeth=Zero
  Square1 : Math  Operator=square  SignedPower=on  RndMeth=Zero
  Square2 : Math  Operator=square  SignedPower=on  RndMeth=Zero
  TRN_Speed : Outport
  wires:
  Demux/1 -> Square/1  "TRN_VelocityX"
  Demux/3 -> Square2/1  "TRN_VelocityZ"
  Demux/2 -> Square1/1  "TRN_VelocityY"
  Square/1 -> Add/1
  Square1/1 -> Add/2
  Square2/1 -> Add/3
  Add/1 -> Sqrt/1
  Sqrt/1 -> TRN_Speed/1
  TRN_VelocityXYZ/1 -> Demux/1

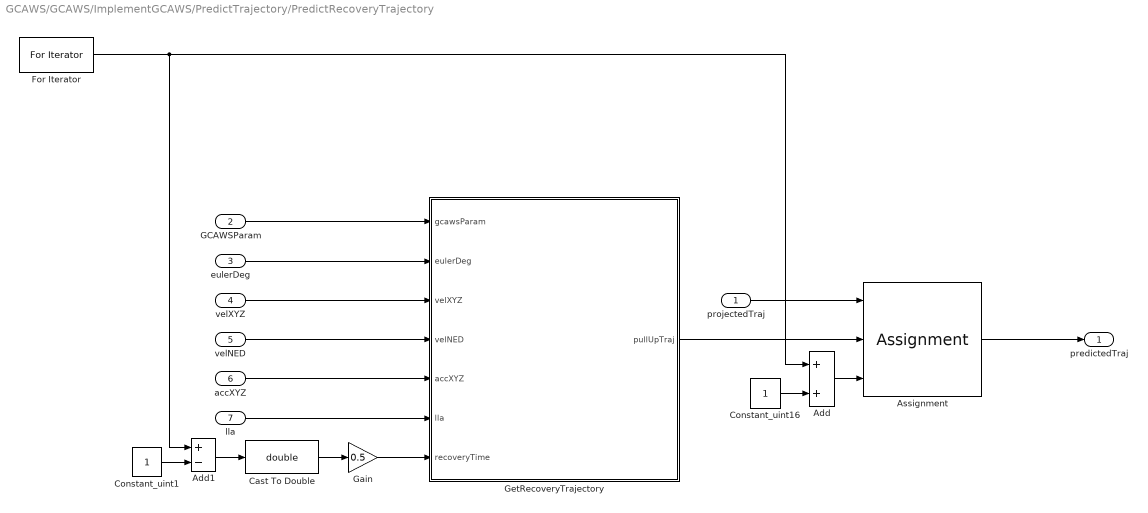
== system GCAWS/GCAWS/ImplementGCAWS/PredictTrajectory/PredictRecoveryTrajectory ==
  projectedTraj : Inport
  GCAWSParam : Inport  Port=2
  eulerDeg : Inport  Port=3
  velXYZ : Inport  Port=4
  velNED : Inport  Port=5
  accXYZ : Inport  Port=6
  lla : Inport  Port=7
  Add : Sum
  Add1 : Sum  Inputs=+-
  Assignment : Assignment  NumberOfDimensions=3  DiagnosticForDimensions=Warning  IndexOptions=Assign all,Index vector (port),Assign all  Indices=1,1,1  OutputSizes=41,12,3
  Cast To Double : DataTypeConversion  OutDataTypeStr=double  SaturateOnIntegerOverflow=off  RndMeth=Floor
  Constant_uint1 : Constant  OutDataTypeStr=uint16
  Constant_uint16 : Constant  OutDataTypeStr=uint16
  For Iterator : ForIterator  IterationLimit=11  IterationVariableDataType=uint16
  Gain : Gain  Gain=0.5
  GetRecoveryTrajectory : MATLAB Function  TreatAsAtomicUnit=on
      settings: RTWSystemCode=Nonreusable function  RTWFcnNameOpts=Use subsystem name  FunctionInterfaceSpec=Allow arguments (Match graphical interface)
  predictedTraj : Outport
  wires:
  GCAWSParam/1 -> GetRecoveryTrajectory/1(gcawsParam)
  eulerDeg/1 -> GetRecoveryTrajectory/2(eulerDeg)
  velXYZ/1 -> GetRecoveryTrajectory/3(velXYZ)
  velNED/1 -> GetRecoveryTrajectory/4(velNED)
  accXYZ/1 -> GetRecoveryTrajectory/5(accXYZ)
  lla/1 -> GetRecoveryTrajectory/6(lla)
  For Iterator/1 -> Add/1, Add1/1
  Assignment/1 -> predictedTraj/1
  projectedTraj/1 -> Assignment/1
  GetRecoveryTrajectory/1(pullUpTraj) -> Assignment/2
  Constant_uint16/1 -> Add/2
  Add/1 -> Assignment/3
  Constant_uint1/1 -> Add1/2
  Add1/1 -> Cast To Double/1
  Cast To Double/1 -> Gain/1
  Gain/1 -> GetRecoveryTrajectory/7(recoveryTime)

== matlab function GCAWS/HandleGCAWSInput/ConfigureReactionTime ==
  data: paramSelected input; reactionTimeSec output; reactionTimeUint16 input
function reactionTimeSec = ConfigureReactionTime(paramSelected, reactionTimeUint16)
%ConfigureReactionTime
% -- INPUT --
% paramSelected	        boolean GCAWS 파라미터 선택 여부		
% reactionTimeUint16    uint16	파일럿 반응시간 
%                               [0.5, 1.0, 1.5(d), 2.0]
% -- OUTPUT
% reactionTimeSec       double  (1) Reaction Time (sec)

% Initialize
reactionTimeSec = 0.0;

% [1] 파일럿 반응시간
if (paramSelected)
    switch reactionTimeUint16
        case uint16(0)
            reactionTimeSec = 0.5;
        case uint16(1)
            reactionTimeSec = 1.0;
        case uint16(2)
            reactionTimeSec = 1.5;
        case uint16(3)
            reactionTimeSec = 2.0;
        otherwise
            reactionTimeSec = 1.5;
    end

else
    % Default
    reactionTimeSec = 1.5;
end

end

== matlab function GCAWS/HandleGCAWSInput/ConfigureMaxPullUpG ==
  data: paramSelected input; maxPullUpG output; pullUpGUint16 input; gsAvailable input; gsAvailableValid input; accZ input
function maxPullUpG = ConfigureMaxPullUpG(paramSelected, pullUpGUint16, gsAvailable, gsAvailableValid, accZ)
%ConfigureMaxPullUpG
% -- INPUT --
% paramSelected	        boolean GCAWS 파라미터 선택 여부
% pullUpGUint16	        uint16	피치축 회복기동에 적용하는 G Onset Rate 
%                               [2.0, 3.0, 4.0(d), 5.0] g/s		
% gsAvailable	        double	현재 허용 가능한 항공기 G		
% gsAvaliableValid	    boolean	현재 허용 가능한 항공기 G의 유효성 플래그		
%
% -- OUTPUT
% maxPullUpG            double  (1) Max Pull Up G (g)

% Initialize
maxPullUpG = 0.0;

% Constants
GRAV_ACC = 9.807;

if (paramSelected)
    switch pullUpGUint16
        case uint16(0)
            maxPullUpG = 3.0;
        case uint16(1)
            maxPullUpG = 3.5;
        case uint16(2)
            maxPullUpG = 4.0;
        case uint16(3)
            maxPullUpG = 5.0;
        otherwise
            maxPullUpG = 4.0;
    end
else
    % Default
    maxPullUpG = 4.0;
end

% G's Available
if gsAvailableValid
    pullUpGTemp = maxPullUpG;
    maxPullUpG = max(-accZ/GRAV_ACC, min(gsAvailable, pullUpGTemp));
else
end

end

== matlab function GCAWS/HandleGCAWSInput/ConfigureRollRate ==
  data: paramSelected input; rollRate output; rollRateUint16 input
function rollRate = ConfigureRollRate(paramSelected, rollRateUint16)
%ConfigureRollRate
% -- INPUT --
% paramSelected	        boolean GCAWS 파라미터 선택 여부
% rollRateUint16        uint16	롤 회복기동 모델에 적용하는 롤 변화율 
%                               [60, 90, 120(d), 150] dps		
% -- OUTPUT --
% rollRate              double  (3) Roll Rate (deg/s)

% Initialize
rollRate = 0.0;

if (paramSelected)
    switch rollRateUint16
        case uint16(0)
            rollRate = 60.0;
        case uint16(1)
            rollRate = 90.0;
        case uint16(2)
            rollRate = 120.0;
        case uint16(3)
            rollRate = 150.0;
        otherwise
            rollRate = 120.0;
    end
else
    % Default
    rollRate = 120.0;
end

end

== matlab function GCAWS/HandleGCAWSInput/ConfigureGOnsetRate ==
  data: paramSelected input; gOnsetRate output; gOnsetRateUint16 input
function gOnsetRate = ConfigureGOnsetRate(paramSelected, gOnsetRateUint16)
%ConfigureGOnsetRate
% -- INPUT --
% paramSelected	        boolean GCAWS 파라미터 선택 여부
% gOnSetRateUint16      uint16	피치축 회복기동에 적용하는 G Onset Rate 
%                               [3.0, 3.5, 4.0(d), 5.0]		
% -- OUTPUT --
% gOnSetRate            double  (4) G-onset rate (g/s)

% Initialize
gOnsetRate = 0.0;

if (paramSelected)
    switch gOnsetRateUint16
        case uint16(0)
            gOnsetRate = 2.0;
        case uint16(1)
            gOnsetRate = 3.0;
        case uint16(2)
            gOnsetRate = 4.0;
        case uint16(3)
            gOnsetRate = 5.0;
        otherwise
            gOnsetRate = 4.0;
    end
else
    % Default
    gOnsetRate = 4.0;
end

end

== matlab function GCAWS/HandleGCAWSInput/ConfigureMaxFlightPath ==
  data: paramSelected input; maxFlightPathAngle output; maxFlightPathUint16 input
function maxFlightPathAngle = ConfigureMaxFlightPath(paramSelected, maxFlightPathUint16)
%ConfigureGOnsetRate
% -- INPUT --
% paramSelected	        boolean GCAWS 파라미터 선택 여부
% maxFlightPathUint16	uint16	회복기동 모델에 적용하는 최대 비행경로각
%                               [45, 60, 75(d), 90] deg
% -- OUTPUT --
% maxFlightPathAngle    double  (5) Max Flight Path Angle (deg)

% Initialize
maxFlightPathAngle = 0.0;

if (paramSelected)
    switch maxFlightPathUint16
        case uint16(0)
            maxFlightPathAngle = 45.0;
        case uint16(1)
            maxFlightPathAngle = 60.0;
        case uint16(2)
            maxFlightPathAngle = 75.0;
        case uint16(3)
            maxFlightPathAngle = 90.0;
        otherwise
            maxFlightPathAngle = 90.0;
    end
else
    % Default
    maxFlightPathAngle = 90.0;
end

end
